simulink model "chap11_1sim"  (R2015a)
settings: Solver=ode45  StartTime=0.0  StopTime=3  RelTol=1e-3
settings Model: Creator=zhr  LastModifiedBy=IT

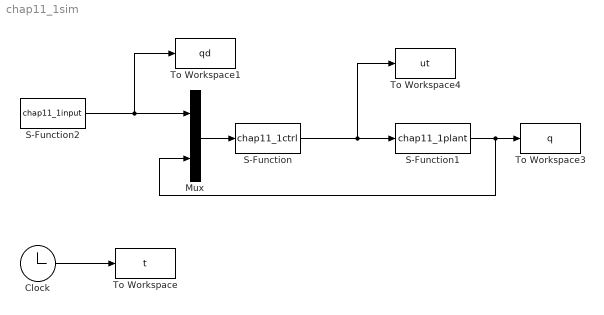
== system chap11_1sim ==
  Clock : Clock
  Mux : Mux  Inputs=2
  S-Function : S-Function  FunctionName=chap11_1ctrl
  S-Function1 : S-Function  FunctionName=chap11_1plant
  S-Function2 : S-Function  FunctionName=chap11_1input
  To Workspace : ToWorkspace  VariableName=t  SampleTime=-1
  To Workspace1 : ToWorkspace  VariableName=qd  SampleTime=-1
  To Workspace3 : ToWorkspace  VariableName=q  SampleTime=-1
  To Workspace4 : ToWorkspace  VariableName=ut  SampleTime=-1
  wires:
  Clock/1 -> To Workspace/1
  Mux/1 -> S-Function/1
  S-Function/1 -> To Workspace4/1, S-Function1/1
  S-Function1/1 -> Mux/2, To Workspace3/1
  S-Function2/1 -> To Workspace1/1, Mux/1
